simulink model "HA_simulation"  (R2024b)
settings: Solver=VariableStepAuto  StartTime=0.0  StopTime=10.0  RelTol=1e-3
settings Model: Creator=Shreesha Kumar  LastModifiedBy=Shreesha Kumar

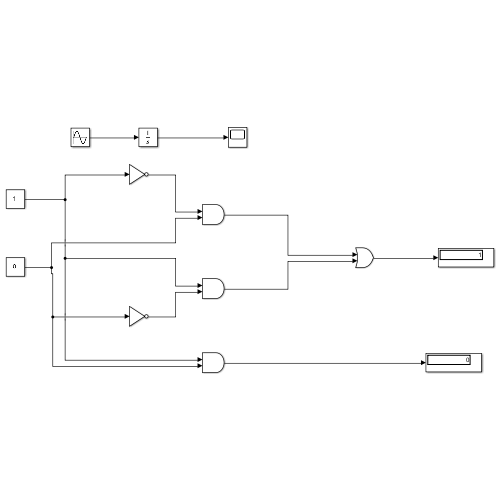
[thumbnail: Simulink's stored preview of the top-level diagram]
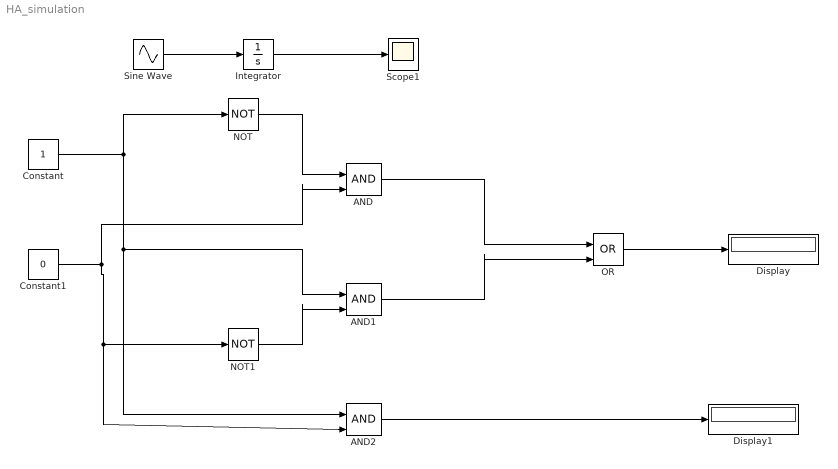
== system HA_simulation ==
  AND : Logic  IconShape=distinctive  AllPortsSameDT=off  OutDataTypeStr=boolean
  AND1 : Logic  IconShape=distinctive  AllPortsSameDT=off  OutDataTypeStr=boolean
  AND2 : Logic  IconShape=distinctive  AllPortsSameDT=off  OutDataTypeStr=boolean
  Constant : Constant
  Constant1 : Constant  Value=0
  Display : Display
  Display1 : Display
  Integrator : Integrator
  NOT : Logic  Operator=NOT  IconShape=distinctive  AllPortsSameDT=off  OutDataTypeStr=boolean
  NOT1 : Logic  Operator=NOT  IconShape=distinctive  AllPortsSameDT=off  OutDataTypeStr=boolean
  OR : Logic  Operator=OR  IconShape=distinctive  AllPortsSameDT=off  OutDataTypeStr=boolean
  Scope1 : Scope
  Sine Wave : Sin  SampleTime=0
  wires:
  Sine Wave/1 -> Integrator/1
  Integrator/1 -> Scope1/1
  NOT/1 -> AND/1
  Constant/1 -> AND2/1, AND1/1, NOT/1
  Constant1/1 -> AND/2, AND2/2, NOT1/1
  NOT1/1 -> AND1/2
  AND/1 -> OR/1
  AND1/1 -> OR/2
  AND2/1 -> Display1/1
  OR/1 -> Display/1
